simulink model "Sim_Modell_RFJ"  (R2020b)
settings: Solver=VariableStepAuto  StartTime=0.0  StopTime=10.0  RelTol=1e-3
undefined symbols (not defined in the file or in its folder): ACD120_80_Rotor, ACD120_80_Stator, Ausleger, Auslegerplatte, DistanzhuelseGP, Federbolzen, Grundplatte, Heidenhain_ERN_1080, Lagerdeckel_oben, Lagerdeckel_unten, par_imp, par_reg, parSys, Seitenplatte, Visualisierung, Welle, X, Y, Z
libraries: sm_lib x37, fl_lib x7, nesl_utility x7, cstblocks x2, simulink x1
(part 3 of 3)

== matlab function Sim_Modell_RFJ/IB-Regler ==
  data: x input; u output; act input; parSys parameter; ML input; par_reg parameter; par_soll input
function u  = fcn(x,act,parSys, ML, par_reg, par_soll)
if(act==0)
    u=0;
else
    
% Zustände
x11 = x(1);
x12 = x(2);
x2  = x(3);

% Reglerparameter -> Parameter_RFJ
k1= par_reg.k1;
gamma=par_reg.gamma1;

% Systemparameter -> Parameter_RFJ
Ia = parSys.I_a;
da = parSys.d_a;
c0 = parSys.c_0;

% Parameter des Sollystems -> Parameter_RFJ
% werden über Simulink eingelesen laut Angabe -> Vorteil?
% par_soll = [par_imp.d, par_imp.M max , par_imp.c]
d    = par_soll(1);
Mmax = par_soll(2);
c    = par_soll(3);

% Rückstellmoment laut Angabe
M = Mmax*tanh(c*x11/Mmax);
d_M_dx11 = c / cosh(c * x11 / Mmax) ^ 2;

% Berechnung der Stellgröße
f1 = [x12 (-c0 * x11 - da * x12 + ML) / Ia]';
g1 = [0 0.1e1 / Ia * c0]';

alpha1 = -(-c0 * x11 + d * x12 - da * x12 + M) / c0;
dalpha1dx1 = [-(-c0 + d_M_dx11) / c0 -(d - da) / c0;];

dV1dx1 = [M - ML Ia * x12;];

u = -k1*(x2-alpha1)-1/gamma*dV1dx1*g1+dalpha1dx1*(f1+g1*x2);
end
end

== matlab function Sim_Modell_RFJ/system (nonlinear)/MATLAB Function ==
  data: x input; omegat input; ML input; xp output
function xp = fcn(x, omegat, ML)
    xp = zeros(3,1);
    xp = RFJ_Student(x, omegat, ML);
end

== matlab function Sim_Modell_RFJ/system (nonlinear)/MATLAB Function1 ==
  data: x input; y output; parSys parameter
function y = fcn(x, parSys)

y = zeros(3,1); % necesary for home

% map the states
phit=x(1);
phia=x(2);
omega=x(3);

% create the output
y(1) = phia;
y(2) = omega;
y(3) = phit;

== matlab function Sim_Modell_RFJ/adaptiv IB-Regler ==
  settings: updateMethod=DISCRETE  sampleTime=par_reg.Ts
  data: x input; u output; act input; parSys parameter; ML_dach_out output; par_reg parameter; par_soll input
function [u,ML_dach_out] = fcn(x,act,parSys, par_reg, par_soll)

    persistent ML_dach
    if isempty(ML_dach) ML_dach = 0; end

    if act==0
    u=0;
    ML_dach = 0;
    ML_dach_out = 0;

    else    %act = 1;
    
    % Zustände übernehmen
    x11 = x(1);
    x12 = x(2);
    x2  = x(3);

    % Reglerparameter -> Parameter_RFJ
    k0 = par_reg.k0;    
    k1= par_reg.k1;
    gamma=par_reg.gamma1;
    Ts = par_reg.Ts;

    % Systemparameter -> Parameter_RFJ
    Ia = parSys.I_a;
    da = parSys.d_a;
    c0 = parSys.c_0;

    % Parameter des Sollystems -> Parameter_RFJ
    % werden über Simulink eingelesen laut Angabe -> Vorteil?
    % par_soll = [par_imp.d, par_imp.M max , par_imp.c]
    d    = par_soll(1);
    Mmax = par_soll(2);
    c    = par_soll(3);

    % Rückstellmoment laut Angabe
    M = Mmax*tanh(c*x11/Mmax);
    dMdx11 = c / cosh(c * x11 / Mmax) ^ 2;

    % Reglerberechnungen ML_dach_out = ML_dach;
    alpha1 = -(-c0 * x11 + d * x12 - da * x12 + M) / c0;
    dalpha1dx1 = [-(-c0 + dMdx11) / c0 -(d - da) / c0;];
    dV1dx1 = [M - ML_dach Ia * x12;];
    f1_dach = [x12 (-c0 * x11 - da * x12 + ML_dach) / Ia]';
    g1 = [0 0.1e1 / Ia * c0]';

    u = -k1*(x2-alpha1)-1/gamma*dV1dx1*g1+dalpha1dx1*(f1_dach+g1*x2);

    % Update des Schätzparameters ML_dach
    dML_dachdt = k0 / Ia * (x2-alpha1) * (d - da) / c0;
    ML_dach = ML_dach + Ts * dML_dachdt;
    ML_dach_out = ML_dach;
    end
end
